simulink model "Copy_of_CM13_2024a_MachE_for_UA_HIL"  (R2024a)
settings: Solver=ode1  StartTime=0.0  StopTime=Inf  FixedStep=0.001  RelTol=1e-3  EnableMultiTasking=on
PreLoadFcn:
  | % if ~length(which('cmcmd')), cmenv; end
PostLoadFcn:
  | if any(exist('dsrtsu_mdlpostloadfcn', 'file') ~= 0), dsrtsu_mdlpostloadfcn('Execute', bdroot); end
InitFcn:
  | , if any(exist('rtifpga_mdlclblib', 'file') ~= 0), rtifpga_mdlclblib('Init', bdroot); end,
  | , if any(exist('dsmpb_private', 'file') ~= 0), dsmpb_private('dsmpb_mdlclblib', 'Init', bdroot); end,
undefined symbols (not defined in the file or in its folder): AccelCmd, ActTqLF_Nm_, ActTqLR_Nm_, ActTqRF_Nm_, ActTqRR_Nm_, BattChargeLimitMaxPwr, BattChargeLimitSocBpts, BattChargeLimitTbl, BattChrgCapcty, BattDischargeLimitSocBpts, BattDischargeLimitTbl, BattDischargeMaxPwr, BattNumCellsParallel, BattNumCellsSeries, BattOpenVoltCapBpts, BattOpenVoltTbl, BattResistSocBpts, BattResistTbl, BattResistTempBpts, BrakeMaxPrs, BrakeMaxTrq, ChassisDistCg2FrontAxle, ChassisDistCg2RearAxle, ChassisVehMass, CltchCmd, CoastDown, DecelCmd, DiffRatio, DiscIntNeverNeededParam, EnvGravCnst, EnvPrs, EnvTemp, FuelSpecificGrav, GearCmd, h, InitStates, lgSw, limitedMCT, MCT, MtrEffSpdBpts, MtrEffTbl, MtrEffTrqBpts, MtrPwrMax, MtrTrqMax, planned_speed, planned_time, pMCT, RealSimPara, ref_speed, Ref_speed, ref_time, Ref_time, rticanmm_blockfcn, rticanmm_initfcn, SteeringCmd, SupvsryCtrlRegenBrkCutOffTbl, SupvsryCtrlRegenSpdBpts, TestScnrioCycleNum, US06, VEH
libraries: simulink x264, VSIGenLib x262, etargetslib x201, dsmpblib x161, CarMaker4SL x142, rtimmsu_dsrtlib x32, vehdynlibtire x24, autolibshared x19, vehdynlibsuspension x14, vehdynlibtirecommon x14, autolibutils x10, VsrLibWheel x8
(part 5 of 47)

== system Copy_of_CM13_2024a_MachE_for_UA_HIL/Vehicle Under Test3/Environment ==
  Grade : Inport
  Friction : Constant  Value=ones(4,1).*1
  Ground Feedback : Subsystem  Variant=on  VariantControlMode=label  LabelModeActiveChoice=0
  Ground Z Level : Constant  Value=zeros(4,1)
  Subsystem : Subsystem
  Subsystem1 : Subsystem
      mask Display: disp('')
  Env : Outport
  wires:
  Subsystem/3(WindVel) -> Subsystem1/3(WindVel)
  Subsystem/2(EnvTemp) -> Subsystem1/2(EnvTemp)
  Subsystem/4(RoadGrade) -> Subsystem1/4(RoadGrade)
  Subsystem/1(EnvPrs) -> Subsystem1/1(EnvPrs)
  Subsystem1/1(Env) -> Env/1
  Friction/1 -> Ground Feedback/1(Friction)
  Ground Feedback/1(Ground) -> Subsystem1/5(GroundBus)  "Gnd"
  Ground Z Level/1 -> Ground Feedback/2(Ground Z Level)
  Grade/1 -> Subsystem/1(Grade)

== system Copy_of_CM13_2024a_MachE_for_UA_HIL/Vehicle Under Test3/Monitor ==
  Monitor : Inport
  Calculate Fuel MPG : Subsystem  Commented=on
  Calculate Powertrain Energy : Subsystem
  Terminator : Terminator
  Terminator3 : Terminator
  wires:
  Calculate Fuel MPG/1(FuelEconMPG) -> Terminator/1  "FuelEconMpg"
  Monitor/1 -> Calculate Powertrain Energy/1(Monitor), Calculate Fuel MPG/1(Monitor)
  Calculate Powertrain Energy/1(TransEnrgyOutkWh) -> Terminator3/1  "DiffEnrgyInkWh"

== system Copy_of_CM13_2024a_MachE_for_UA_HIL/Vehicle Under Test3/Performance Calculations ==
  VehSpd : Inport
  BattPwr : Inport  Port=2
  Divide : Product  Inputs=*/
  Divide1 : Product  Inputs=*/
  Divide2 : Product  Inputs=*/
  Integrator : Integrator
  Integrator1 : Integrator
  L/100 Km Calc : Product  Inputs=/*
  Product : Product
  Rate Transition3 : RateTransition  Deterministic=off
  Saturation : Saturate  UpperLimit=Inf  LowerLimit=0.001
  Saturation1 : Saturate  UpperLimit=Inf  LowerLimit=1e-3
  Sqrt : Sqrt
  US EPA kwh/USgal equivalent : Constant  Value=33.7
  US MPG Calc : Product  Inputs=*/
  m to 100Km : Gain  Gain=1/1000/100
  m to mile : Gain  Gain=0.000621371
  m^3 per gal : Gain  Gain=0.00378541
  m^3 to L : Gain  Gain=1000
  m^3 to US Gal : Gain  Gain=264.172
  s per h : Constant  Value=3600
  w per kw : Constant  Value=1000
  US MPG : Outport  VectorParamsAs1DForOutWhenUnconnected=off
  L/100Km : Outport  Port=2  VectorParamsAs1DForOutWhenUnconnected=off
  wires:
  VehSpd/1 -> Product/1, Product/2
  Product/1 -> Sqrt/1
  Sqrt/1 -> Integrator/1
  BattPwr/1 -> Divide/1
  US EPA kwh/USgal equivalent/1 -> Divide2/2
  m^3 per gal/1 -> Integrator1/1
  Divide1/1 -> m^3 per gal/1
  s per h/1 -> Divide1/2
  Divide2/1 -> Divide1/1
  Divide/1 -> Divide2/1
  w per kw/1 -> Divide/2
  Rate Transition3/1 -> US MPG/1  "US MPG"
  Saturation1/1 -> US MPG Calc/2
  US MPG Calc/1 -> Rate Transition3/1
  L/100 Km Calc/1 -> L/100Km/1  "L/100Km"
  m to 100Km/1 -> Saturation/1
  Saturation/1 -> L/100 Km Calc/1
  Integrator1/1 -> m^3 to L/1, m^3 to US Gal/1
  m to mile/1 -> US MPG Calc/1
  Integrator/1 -> m to 100Km/1, m to mile/1
  m^3 to L/1 -> L/100 Km Calc/2
  m^3 to US Gal/1 -> Saturation1/1

== system Copy_of_CM13_2024a_MachE_for_UA_HIL/Vehicle Under Test3/Vehicle ==
  note: With tire radius correction of 1.14
  note: NOT USED
  note: Vehicle simulation type:
      | 0- Simulink offline model
      | 1- Rototest HIL model
  note: NOT USED
  Env : Inport
  Driver : Inport  Port=2
  CarCmd : Inport  Port=3
  Abs : Abs  Commented=on  SaturateOnIntegerOverflow=off
  Actuation and Outputs : Subsystem
  AxT : Scope
  AxT2 : Scope  Commented=on
  Battery : Subsystem
  Bus Creator : BusCreator  Inputs=6
  Bus Selector : BusSelector  OutputSignals=Omega
  Bus Selector1 : BusSelector  Commented=on  OutputSignals=BRAKE_LAMP_BOOL_CAN,STEERING_ANGLE_DEG_CAN
  Bus Selector2 : BusSelector  Commented=on  OutputSignals=CarTrqT2W,VehSpd,Fx
  Bus Selector3 : BusSelector  Commented=on  OutputSignals=PT IF WFL rotv,PT IF WFR rotv,PT IF WRL rotv,PT IF WRR rotv
  Constant : Constant  Commented=on  Value=0  SampleTime=-1
  Data Type Conversion : DataTypeConversion  Commented=on  SaturateOnIntegerOverflow=off  RndMeth=Floor
  Data Type Conversion1 : DataTypeConversion  Commented=on  SaturateOnIntegerOverflow=off  RndMeth=Floor
  DriveCycle_trigger : Constant  Value=0
  Driver and Drive Cycle : Subsystem  TreatAsAtomicUnit=on
  From CAN : Subsystem  Commented=on
  From10 : From  Commented=on  GotoTag=VehSpdKph
  Front Wheel Drive : Subsystem  Variant=on  VariantControlMode=label  VariantControl=1  LabelModeActiveChoice=Choice
  Gain : Gain  Gain=3.6
  Gain1 : Gain  Commented=on  Gain=3.6*1.1414
  Goto10 : Goto  Commented=on  GotoTag=VehSpdKph
  Goto7 : Goto  Commented=on  GotoTag=BrakePressedCAN
  Goto8 : Goto  Commented=on  GotoTag=SteeringCAN
  Motor : Subsystem
  MtT : Scope
  MtT1 : Scope
  Multiport Switch : MultiPortSwitch  DataPortOrder=Zero-based contiguous  Inputs=2  zeroidx=on  SaturateOnIntegerOverflow=off  InputSameDT=off
  "Powertrain Supervisory Controller " : Subsystem  AncestorBlock=LibPtSupervisoryCtrl/Powertrain Supervisory Controller
  "Rototest UDP RX ExternalMode  " : Subsystem  Commented=on
  "Rototest UDP TX ExternalMode  " : Subsystem  Commented=on
  Rototest and ORNL Interface : Subsystem  Commented=on
  SUMO_speed_level : Constant  Value=0
  Scope : Scope
  Switch : Switch  Commented=on  Threshold=0.1  SaturateOnIntegerOverflow=off  InputSameDT=off
  Terminator{,1..2,4} (4 alike) : Terminator  Commented=on
  Terminator3 : Terminator
  To Workspace1 : ToWorkspace  VariableName=rotoOmega1  SampleTime=-1
      settings: Save2DSignal=2-D array (concatenate along first dimension)
  To Workspace2 : ToWorkspace  Commented=on  VariableName=rotoOmega  SampleTime=-1
      settings: Save2DSignal=2-D array (concatenate along first dimension)
  Transfer Fcn{,1..3} (4 alike) : TransferFcn  Commented=on  Denominator=[0.01 1]
  Transfer Fcn12 : TransferFcn  Commented=on  Denominator=[0.02 1]
  Vector Concatenate : Concatenate  Commented=on  NumInputs=4
  Vehicle Dynamics : Subsystem  Variant=on  VariantControlMode=label  LabelModeActiveChoice=Veh14DOF  mask{VehDynSel=Vehicle 14DOF}
      mask prompts: VehDynSel "Select the driver"
      mask init: same as Copy_of_CM13_2024a_MachE_for_UA_HIL/Vehicle Under Test2/Vehicle/Vehicle Dynamics
      mask TypeOptions VehDynSel: Vehicle Longitudinal | Vehicle 7DOF | Vehicle 14DOF
  VehicleSimulationType : Constant  Value=0
  omega : Scope
  Veh : Outport
  Output : Outport  Port=2
  wires:
  "Powertrain Supervisory Controller "/1(SupvsryCtrl) -> Vehicle Dynamics/2(SupvsryCtrl), Motor/1(SupvsryCtrl), [SupvsryCtrl]
  Driver/1 -> "Powertrain Supervisory Controller "/1(Driver)
  Bus Creator/1 -> Veh/1  "Veh"
  [SupvsryCtrl] -> Bus Creator/1  "SupvsryCtrl"
  [Batt] -> Bus Creator/2  "Batt"
  [Mtr] -> Bus Creator/3  "Mtr"
  [Whl] -> Bus Creator/5  "Whl"
  [Chassis] -> Bus Creator/6  "Chassis"
  Battery/1(Batt) -> [Batt], "Powertrain Supervisory Controller "/4(Batt)
  Motor/1(Mtr) -> "Powertrain Supervisory Controller "/3(Mtr), [Mtr]
  Env/1 -> Vehicle Dynamics/1(Env)
  Vehicle Dynamics/2(Chassis) -> "Powertrain Supervisory Controller "/2(Chassis), [Chassis]
  Vehicle Dynamics/1(Whl) -> [Whl]
  [Whl] -> Bus Selector/1
  [Diff] -> Bus Creator/4  "Diff"
  Front Wheel Drive/1(Diff) -> [Diff]
  Front Wheel Drive/3(PropShaftSpd) -> MtT1/1, Motor/2(MtrSpd)
  Motor/2(MtrTrq) -> Front Wheel Drive/1(DrvShfTrq), MtT/1
  Front Wheel Drive/2(AxlTrq) -> AxT/1, Vehicle Dynamics/3(AxlTrq)
  Rototest and ORNL Interface/2(Powertrain Out) -> Bus Selector3/1, Terminator/1
  Rototest and ORNL Interface/4(WhlSpd) -> To Workspace2/1, Terminator4/1  "WhlSpdCmd"
  Vehicle Dynamics/3(RototestInput) -> [RototestInput]
  VehicleSimulationType/1 -> Multiport Switch/1
  Driver and Drive Cycle/1(DriverBus) -> Actuation and Outputs/1(Driver Commands)
  Bus Selector1/1 -> Data Type Conversion1/1  "<BRAKE_LAMP_BOOL_CAN>"
  Data Type Conversion/1 -> Goto8/1  "SteerAngleCAN"
  "Rototest UDP RX ExternalMode  "/1(Data Vector) -> Rototest and ORNL Interface/2(UDP Input)
  Data Type Conversion1/1 -> Rototest and ORNL Interface/3(BRAKE_PRESSED), Goto7/1, Terminator2/1  "BrakePressed_flag"
  Bus Selector1/2 -> Data Type Conversion/1  "<STEERING_ANGLE_DEG_CAN>"
  From CAN/1(IO_Out) -> Bus Selector1/1
  Actuation and Outputs/1(BrakeSwitch) -> From CAN/1(BrakeSwitch)
  Actuation and Outputs/2(CAVE_Driver) -> Terminator3/1  "CAVE_Driver_Cmd"
  Rototest and ORNL Interface/3(DataSend) -> "Rototest UDP TX ExternalMode  "/1(Rototest_UDP_TX)  "Rototest_UDP_TX"
  Rototest and ORNL Interface/1(BrakeUpd) -> Terminator1/1
  [RototestInput] -> Bus Selector2/1
  Bus Selector2/3 -> Rototest and ORNL Interface/5(FXIN)  "<Fx>"
  Bus Selector2/2 -> Transfer Fcn12/1  "<VehSpd>"
  Bus Selector2/1 -> Rototest and ORNL Interface/1(CarTrqT2W)  "<CarTrqT2W>"
  Bus Selector/1 -> Multiport Switch/2  "<Omega>"
  Bus Selector3/1 -> Transfer Fcn/1  "<PT IF WFL rotv>"
  Bus Selector3/2 -> Transfer Fcn1/1  "<PT IF WFR rotv>"
  Bus Selector3/3 -> Transfer Fcn2/1  "<PT IF WRL rotv>"
  Bus Selector3/4 -> Transfer Fcn3/1  "<PT IF WRR rotv>"
  Vector Concatenate/1 -> Scope/1, To Workspace1/1, [OmegaRoto]
  [OmegaRoto] -> Multiport Switch/3
  Gain1/1 -> AxT2/1, Rototest and ORNL Interface/4(vehSpeedKph), Goto10/1  "VehSpdKph"
  Gain/1 -> Driver and Drive Cycle/1(Veh speed feedback [kph])
  DriveCycle_trigger/1 -> Driver and Drive Cycle/2(Veh speed cycle trigger)
  Multiport Switch/1 -> Front Wheel Drive/2(Omega), omega/1
  Constant/1 -> Switch/3
  Switch/1 -> Gain1/1
  Abs/1 -> Switch/2
  Transfer Fcn/1 -> Vector Concatenate/1
  Transfer Fcn1/1 -> Vector Concatenate/2
  Transfer Fcn2/1 -> Vector Concatenate/3
  Transfer Fcn3/1 -> Vector Concatenate/4
  Transfer Fcn12/1 -> Switch/1, Abs/1
  CarCmd/1 -> Actuation and Outputs/2(CarlaGBS), Driver and Drive Cycle/4(CarlaRef)
  Driver and Drive Cycle/2(Output) -> Output/1
  SUMO_speed_level/1 -> Driver and Drive Cycle/3(SUMO Veh speed Cmd Level)
  [vehSpeedSim] -> Gain/1
  connections:
  Battery/RConn1 -- Motor/LConn1

== system Copy_of_CM13_2024a_MachE_for_UA_HIL/CarMaker/IPG Vehicle/AEB Flag ==
  Bus Selector : BusSelector  OutputSignals=ACCDATA_2.CmbbBrkDecel_A_Rq,PowertrainData_10.TrnRng_D_Rq,PowertrainData_10.TrnPrkSys_D_Actl,PowertrainData_10.GearPos_D_Actl,PowertrainData_10.GearLvr_D_ActlDrv,Battery_Traction_2_FD1.BattTrac_U2_Actl,Battery_Traction_2_FD1.BattTrac_I2_Actl
  Gain{,1..4,6} (6 alike) : Gain
  RTICANMM ControllerSetup : Subsystem  InitFcn=rticanmm_blockfcn('InitFcn', 'CANnedySetup', gcb)  ClipboardFcn=rticanmm_blockfcn('ClipboardFcn', 'CANnedySetup', gcb)  mask(RTICANMM){DSProperties=struct('RTI',struct('Version',uint32(1),'BlockType',struct('isSLSource',uint8(1),'isSLSink',uint8(1),'isHWSource',uint8(0),'isHWSink',uint8(0),'isSetup',uint8(0),'isInline',uint8(1),'isNonInline',uint8(0),'isInterrupt',uint8(0),'isChannelwise',uint8(0)),'IOBoardType','RTICANMM','UnitType','RTICANMM','Identifier','BUSSETUP','DialogType','SL','BlockSet','RTICANMM','SlaveProcessor','CAN')), CANMMProperties=struct('cannedy',struct('data',struct('options',struct('controllername','MachE_FD1','controllernameautomatic',0,'loglevel','0','checkrealtime',0,'checkchangebaudrate',0,'sampletime','1.000','CANControllerStatus',1,'NumberofStuffErr',0,'NumberofFormErr',0,'NumberofAckErr',0,'NumberofBit0Err',1,'NumberofsuccrecRX',0,'Numberofsuccsent',0,'NumberofBit1Err',1,'NumberofCRCErr',1,'NumberoflostRX',0,'Busoff',0,'Busload',0,'OperationPending',0,'TxRetryCount',3,'addtrcexclusion',true,'cannavigator',struct('checkmonitoring',0,'checkinternmonitoring',0),'show_usrtrc',0,'use_usrtrc',0,'checkchangebaudrateFD',0,'errorframegeneration',0,'efgenabled',1),'modelroot','C:\GitDev\Yunli\FordMachE\HIL-Operation\src_cm4sl','generalsettings',struct('setupdata',struct('board','DS2671','boardno',1,'channelno',1,'Type','STD','transceiver',['ISO 11898-2 HIGH SPEED CAN'],'busconfig',[],'feedthrough','false','resistance',struct('r120',1,'roff',0,'r16',0,'r10',1),'baudrate','500','Frequency',[24 36],'samplemode',1,'commChannelTJA1041',6,'config',struct('standard',1,'advanced',0,'register',struct('btr0','0xC0','btr1','0x6F','sp','70','sjw','v','tseg1','15','tseg2','6','brp','0','smpl','0','btr0_36','0x1','btr1_36','0x2D','sp_36','83','sjw_36','0','tseg1_36','12','tseg2_36','2','brp_36','1','smpl_36','0','btr0_64','0x3','btr1_64','0x2B','sp_64','81','sjw_64','0','tseg1_64','11','tseg2_64','2','brp_64','3','smpl_64','0')),'channelcfg',struct('INTENDISABLE','CAN_INT_DISABLE','intenable',0),'SETUPID','RTICANMM_MachE_FD1_ID','CONTROLLER_ID','CANMM_CTL_SETUP_MachE_FD1','mainblock_includefile','RTICANMM_SETUP_MachE_FD1','canfdenable',2,'canfdboardselected',1,'slotno',1,'moduletype','DS4342','baudrateFD','2000','samplePoint','80','samplePointFD','80','termination','TERMINATION_ON'),'filesettings',struct('destfolder',struct('Name','RTICANMM_FILES','Check',1),'buildfolder',struct('Name','.','Check',1))),'advanced',struct('options',ones(1,100)),'partialnetdata',struct('switchedon',0,'format','STD','idmask',['XXXXX XXXXXXXX XXXXXXXX XXXXXXXX'],'idcode','0','idfilter','0','datamaskused',0,'datalength','0','datamask','0x0000000000000000','partialnetworkenable',0)),'blk',['HIL_MachE_CM10/Vehicle Under Test/Vehicle/AEB Flag/RTICANMM' char(10) 'ControllerSetup'],'allgeneratedfiles',{{'C:\GitDev\Yunli\FordMachE\HIL-Operation\src_cm4sl\RTICANMM_FILES\RTICANMM_SETUP_MachE_FD1.c','C:\GitDev\Yunli\FordMachE\HIL-Operation\src_cm4sl\RTICANMM_FILES\RTICANMM_SETUP_MachE_FD1.h','c:\gitdev\yunli\fordmache\hil-operation\src_cm4sl\rticanmm_files\rticanmm_setup_mache_fd1.mexw64'}},'ismp',false,'BlockDataVersion','0.9.0','recreate',0,'CANnedyTag','MachE_FD1'),'CANnedynew',0,'CANnedySettings','MachE_FD1','GeneratedFiles',{{'C:\GitDev\Yunli\FordMachE\HIL-Operation\src_cm4sl\RTICANMM_FILES\RTICANMM_SETUP_MachE_FD1.c','C:\GitDev\Yunli\FordMachE\HIL-Operation\src_cm4sl\RTICANMM_FILES\RTICANMM_SETUP_MachE_FD1.h','c:\gitdev\yunli\fordmache\hil-operation\src_cm4sl\rticanmm_files\rticanmm_setup_mache_fd1.mexw64'}},'SFCN','RTICANMM_SETUP_MachE_FD1.c','HostService',struct('Tags',struct('DATA','RTICANMM_MonitorData','TimeStampGlobal','RTICANMM_MonitoringTimeStamp','TimeStampGlobalEnable','RTICANMM_MonitoringTimeStampEnable','Enable','CANMMMonitor_MachE_FD1','TimeStamp','MonitoringTimeStamp_MachE_FD1'),'DATA',struct('Length',18),'Info',struct('Desc',{'ID','Service','Data1','Data2','Data3','Data4','Data5','Data6','Data7','Data8','Data9','Data10','Data11','Data12','Data13','Data14','Data15','Data16'}),'Names',struct('TimeStampGlobal','TimeStamp','TimeStampGlobalEnable','TimeStamp_Enable','Enable','Monitoring_Enable','TimeStamp','Monitoring_TimeStamp'),'ChannelID',2)), CANMMType=CANnedySetup, CANMMFolder=C:\CM_Projects\UA_cave\CM13_proj\src_cm4dspace_realsim, CANMMDestFolder=RTICANMM_FILES, CANMMSettings=MachE_FD1, CANMMSFcn=RTICANMM_SETUP_MachE_FD1, CANMMBoard=DS2671, CANMMBoardNum=1, CANMMChannel=1}
      settings: AttributesFormatString=%<CANMMSettings>  CopyFcn=rticanmm_blockfcn('CopyFcn', 'CANnedySetup', gcb)  DeleteFcn=rticanmm_blockfcn('DeleteFcn', 'CANnedySetup', gcb)  ModelCloseFcn=rticanmm_blockfcn('ModelCloseFcn', 'CANnedySetup', gcb)  NameChangeFcn=rticanmm_blockfcn('NameChangeFcn', 'CANnedySetup', gcb)  OpenFcn=try, rticanmm_setup_gui('create',gcb); ; catch,errordlg({lasterr, '','Please check your RTI installation.'},['Error: ' upper(bdroot)], 'replace'); end  MoveFcn=rticanmm_blockfcn('MoveFcn', 'CANnedySetup', gcb)
      mask Help: eval('rticanmm_quickstart(''create'', gcb);', 'disp(lasterr);')
      mask Display:
      | disp('RTI CAN\nMultiMessage\nControllerSetup')
      | 
      | port_label('input', 1 , 'Variation')
      | port_label('input', 2 , 'Reset')
      | port_label('output', 1, 'Status')
      | port_label('output', 2, 'Bit 0 errors')
      | port_label('output', 3, 'Bit 1 errors')
      | port_label('output', 4, 'CRC errors')
  RTICANMM ControllerSetup1 : dsmpblib/Data Outport  Priority=-10000
      settings: SourceProductName=dSPACE Model Interface Package for Simulink (MIPS)
  RTICANMM MainBlock : Subsystem  InitFcn=rticanmm_blockfcn('InitFcn', 'CANnedy', gcb)  ClipboardFcn=rticanmm_blockfcn('ClipboardFcn', 'CANnedy', gcb)  mask(RTICANMM){DSProperties=struct('RTI',struct('Version',uint32(1),'BlockType',struct('isSLSource',uint8(1),'isSLSink',uint8(1),'isHWSource',uint8(0),'isHWSink',uint8(0),'isSetup',uint8(0),'isInline',uint8(1),'isNonInline',uint8(0),'isInterrupt',uint8(0),'isChannelwise',uint8(0)),'IOBoardType','RTICANMM','UnitType','RTICANMM','Identifier','Mainblock','DialogType','SL','BlockSet','RTICANMM','SlaveProcessor','CAN')), CANMMProperties=struct('RTICANMMVersion','24.1','RTICANMMVersionIntern','24.1.739338.0305092592','RTICANMMDate','02-May-2024','Settings','RTICANMM_MAIN_MachE_FD1','UserTracePath','','ModelPath','C:\CM_Projects\UA_cave\CM13_proj\src_cm4dspace_realsim','filesettings',struct('FileName','RTICANMM_FILES\FD1_CAN_CX727_BEV_MY21_DCV_V21.dbc','IsRelative',1,'ClusterId',1,'ClusterList',{{'default'}},'destfolder',struct('Name','RTICANMM_FILES','Check',1),'buildfolder',struct('Name','.','Check',1),'onlyfreerawcapture',0,'overlapping2variant',0,'canfdsupport',1,'shortestJ2container',1),'onlyfreerawcapture',0,'Board','DS2671','BoardNum','1','ChannelNum','1','Variation','1','SetupId','MachE_FD1','MARK',['1F517A29CDDA91C40D81A06F1A259F';'402B427622E552C8724AFAF21BAF37';'507793A5241270CA8226E0AA5FABF0';'03D6615B00574698D00C6826B10C14';'3DF76DA45C804484AF6D3344981453'],'date','08-May-2025','clock',['08.05.2025 17:13:54'],'recreate',0,'RTIVER','DSRT','j1939',0,'TRC',struct('include',1),'rtsupport',struct('XMLFile','C:\CM_Projects\UA_cave\CM13_proj\src_cm4dspace_realsim\RTICANMM_FILES\RTICANMM_MAIN_MachE_FD1.xml','DBCXML',struct('Path','C:\CM_Projects\UA_cave\CM13_proj\src_cm4dspace_realsim\RTICANMM_FILES\RTICANMM_MAIN_MachE_FD1_dbc.xml','support',1,'Name','FD1_CAN_CX727_BEV_MY21_DCV_V21.dbc','Date',['28-Mar-2023 17:18:35'],'Type','CAN_FD','DBCSupport','ON'))), CANMMType=CANnedy, CANMMUserTraceMerged=off, CANMMUserTracePath=, CANMMChannelNum=1, CANMMBoardNum=1, CANMMDestFolder=RTICANMM_FILES, CANMMFolder=., CANMMSetupId=MachE_FD1, CANMMsave2mat=['1F517A29CDDA91C40D81A06F1A259F';'402B427622E552C8724AFAF21BAF37';'507793A5241270CA8226E0AA5FABF0';'03D6615B00574698D00C6826B10C14';'3DF76DA45C804484AF6D3344981453'], CANMMName=MachE_FD1, CANMMSettings=RTICANMM_MAIN_MachE_FD1, CANMMIntermediateTag=RTICANMM_MAIN_MachE_FD1_intermediate, CANMMsfcnname=RTICANMM_MAIN_MachE_FD1}
      mask init:
      | rticanmm_initfcn(gcb, CANMMType, CANMMsfcnname)
      settings: AttributesFormatString=MachE_FD1[MachE_FD1]  CopyFcn=rticanmm_blockfcn('CopyFcn', 'CANnedy', gcb)  DeleteFcn=rticanmm_blockfcn('DeleteFcn', 'CANnedy', gcb)  ModelCloseFcn=rticanmm_blockfcn('ModelCloseFcn', 'CANnedy', gcb)  NameChangeFcn=rticanmm_blockfcn('NameChangeFcn', 'CANnedy', gcb)  OpenFcn=try, rticanmm_main_gui('create',gcb); ; catch,errordlg({lasterr, '','Please check your RTI installation.'},['Error: ' upper(bdroot)], 'replace'); end  MoveFcn=rticanmm_blockfcn('MoveFcn', 'CANnedy', gcb)
      mask Help: try, rticanmm_quickstart('create', gcb); catch ME, disp(ME.message);end
      mask Display:
      | disp(sprintf('RTI CAN\nMultiMessage\nMainBlock'))
      | port_label('output', 1, 'RX Data')
  Reset@RTICANMM ControllerSetup : Constant  Value=0  OutDataTypeStr=boolean
  Terminator{,1..6,9..11} (10 alike) : Terminator
  Variation@RTICANMM ControllerSetup : Constant  OutDataTypeStr=uint8
  Output : Outport
  wires:
  Variation@RTICANMM ControllerSetup/1 -> RTICANMM ControllerSetup/1(VariationInput)
  Reset@RTICANMM ControllerSetup/1 -> RTICANMM ControllerSetup/2(Reset)
  Bus Selector/1 -> Output/1  "<CmbbBrkDecel_A_Rq>"
  Bus Selector/2 -> Gain4/1  "<TrnRng_D_Rq>"
  RTICANMM ControllerSetup/1(BUS_STATE) -> Terminator1/1  "FD1_status"
  RTICANMM ControllerSetup/2(STATUS_BIT0_ERROR) -> Terminator2/1  "FD1_bit0_err"
  RTICANMM ControllerSetup/3(STATUS_BIT1_ERROR) -> Terminator3/1  "FD1_bit1_err"
  RTICANMM ControllerSetup/4(STATUS_CRC_ERROR) -> Terminator4/1  "FD1_CRC_err"
  Bus Selector/3 -> Gain3/1  "<TrnPrkSys_D_Actl>"
  Bus Selector/6 -> Gain2/1  "<BattTrac_U2_Actl>"
  Bus Selector/7 -> Gain1/1  "<BattTrac_I2_Actl>"
  Bus Selector/4 -> Gain/1  "<GearPos_D_Actl>"
  Bus Selector/5 -> Gain6/1  "<GearLvr_D_ActlDrv>"
  Gain4/1 -> Terminator6/1  "GearPos_D_Actl"
  Gain3/1 -> Terminator5/1  "GearPos_D_Actl"
  Gain/1 -> Terminator/1  "GearPos_D_Actl"
  Gain6/1 -> Terminator11/1  "GearLvr_D_Actl"
  Gain2/1 -> Terminator10/1  "BattTrac_U2_Actl"
  Gain1/1 -> Terminator9/1  "BattTrac_I2_Actl"
  RTICANMM MainBlock/1(RX_Data) -> Bus Selector/1

== system Copy_of_CM13_2024a_MachE_for_UA_HIL/CarMaker/IPG Vehicle/Actuation and Outputs ==
  note: Notes: 11.12.2024
      | Increased the brake limite from 50 to 80
  note: CarMaker Driver's Brake value is too mall to hold the Mach-E when parking
      | Instead of default value, we change it to 40%
  note: Pedal Control Selection
      | 1. Manual input
      | Gas: percentage
      | Brake: percentage
      | 2. From Driver bus commands
      | 3. CM Driver
      | 4. 0
  note: Temp added an Soft_AEB for testing
  note: Detect Rising signal from M_SW_signal.
      | When SW is turned on, reset AEB flag
  note: Driver Commands are [0,100] for both pedal and brake
  Driver Commands : Inport
  CM Driver Commands : Inport  Port=2
  AEB Cmd : Inport  Port=3
  A_M_SW_Sig : Inport  Port=4
  Veh_spd : Inport  Port=5
  AEB Flag Control : Logic  Operator=OR  IconShape=distinctive  AllPortsSameDT=off  OutDataTypeStr=boolean
  AND : Logic  IconShape=distinctive  AllPortsSameDT=off  OutDataTypeStr=boolean
  APP : Constant  Value=0
  AR_limit : Saturate  UpperLimit=100  LowerLimit=0
  Add : Sum
  Add1 : Sum
  BR_command_0to100 : Constant  Value=0
  BR_limit : Saturate  UpperLimit=80  LowerLimit=0
  Bus Creator : BusCreator  Inputs=2
  Bus Selector : BusSelector  Commented=on  OutputSignals=VhclCtrl Gas
  Bus Selector1 : BusSelector  OutputSignals=AccelPedalCmd
  Bus Selector2 : BusSelector  Commented=on  OutputSignals=VhclCtrl Brake
  Bus Selector3 : BusSelector  OutputSignals=BrakePedalCmd
  Compare To Constant : simulink/Logic and Bit Operations/Compare To Constant  relop=>=  const=3  OutDataTypeStr=boolean
  Compare To Constant1 : simulink/Logic and Bit Operations/Compare To Constant  relop=<=  const=0.1  OutDataTypeStr=boolean  ZeroCross=off
  Compare To Constant2 : simulink/Logic and Bit Operations/Compare To Constant  relop=<=  const=0.01  OutDataTypeStr=boolean  ZeroCross=off
  Constant : Constant  Value=0
  Constant1 : Constant  Value=0
  Constant2 : Constant  Value=0
  Detect Rise Positive : simulink/Logic and Bit Operations/Detect Rise Positive  vinit=0  OutDataTypeStr=boolean
  Gain : Gain  Gain=-1
  Gain1 : Gain  Gain=100
  Gain2 : Gain  Gain=100
  MOOG Brake Actuator : Subsystem
  Memory : Memory
  Min threshold for Brake switch : Constant  Value=0
  Multiport Switch1 : MultiPortSwitch  Inputs=4  SaturateOnIntegerOverflow=off  InputSameDT=off
  Multiport Switch2 : MultiPortSwitch  Inputs=4  SaturateOnIntegerOverflow=off  InputSameDT=off
  Pedal Reset : Constant  Value=0
  Pedal Robot Control Selection : Constant  Value=2
  Relational Operator : RelationalOperator  Operator=>  OutDataTypeStr=boolean  InputSameDT=off
  Soft_AEB : Constant  Value=0
  Switch : Switch  Criteria=u2 > Threshold  SaturateOnIntegerOverflow=off  InputSameDT=off
  Switch1 : Switch  Criteria=u2 > Threshold  SaturateOnIntegerOverflow=off  InputSameDT=off
  Switch4 : Switch  Criteria=u2 > Threshold  SaturateOnIntegerOverflow=off  InputSameDT=off
  Terminator : Terminator
  Vehicle Accel Pedal Voltage Output : Subsystem
  bped2br_N1 : Lookup_n-D  NumberOfTableDimensions=1  BreakpointsForDimension1=[0 0.1 0.2 100]  Table=[0 0 25 100]  InternalRulePriority=Speed  RndMeth=Simplest
  standstill brake [0,100] : Constant  Value=0.4
  BrakeSwitch : Outport  VectorParamsAs1DForOutWhenUnconnected=off
  CAVE_Driver : Outport  Port=2
  AEB_IS_Triggered : Outport  Port=3
  tag scope: BrakeDriver=global, CarlaSteer=global, GasDriver=global
  wires:
  Multiport Switch1/1 -> AR_limit/1
  APP/1 -> Multiport Switch1/2
  Bus Selector1/1 -> Multiport Switch1/3  "<AccelPedalCmd>"
  Gain2/1 -> Multiport Switch1/4
  Multiport Switch2/1 -> BR_limit/1
  Gain1/1 -> Multiport Switch2/4
  Driver Commands/1 -> Bus Selector3/1, Bus Selector1/1
  Pedal Robot Control Selection/1 -> Multiport Switch1/1, Multiport Switch2/1
  BR_command_0to100/1 -> Multiport Switch2/2
  CM Driver Commands/1 -> Bus Selector2/1, Bus Selector/1
  Bus Selector3/1 -> Multiport Switch2/3  "<BrakePedalCmd>"
  Min threshold for Brake switch/1 -> Relational Operator/2
  Relational Operator/1 -> BrakeSwitch/1  "BrakeSwitch"
  Constant/1 -> Multiport Switch1/5
  Constant1/1 -> [CarlaSteer], Multiport Switch2/5
  Bus Creator/1 -> CAVE_Driver/1
  BR_limit/1 -> MOOG Brake Actuator/1(Brake Pedal command [%]), Bus Creator/2, [BrakeDriver], Relational Operator/1  "BrakePedalCmd_pct"
  Switch/1 -> Vehicle Accel Pedal Voltage Output/1(APP_pct), [GasDriver], Bus Creator/1  "AccelPedalCmd_pct"
  Constant2/1 -> Switch1/1, Switch/1
  AEB Cmd/1 -> Gain/1
  Add/1 -> Memory/1
  Compare To Constant/1 -> Add1/2
  AR_limit/1 -> Switch/3  "AccelPedalCmd_pct"
  Gain/1 -> Compare To Constant/1
  Switch1/1 -> Add/2  "AccelPedalCmd_pct"
  Pedal Reset/1 -> AEB Flag Control/2
  Memory/1 -> AEB_IS_Triggered/1, Switch/2, Switch1/3
  A_M_SW_Sig/1 -> Detect Rise Positive/1
  Detect Rise Positive/1 -> AEB Flag Control/1
  AEB Flag Control/1 -> Terminator/1, Switch1/2  "AEB Flag Control"
  Soft_AEB/1 -> Add1/1
  Add1/1 -> Add/1
  standstill brake [0,100]/1 -> Switch4/1
  Compare To Constant1/1 -> AND/2
  Bus Selector2/1 -> Switch4/3  "<VhclCtrl Brake>"
  Switch4/1 -> Gain1/1  "BrakePedalPos_pct"
  Veh_spd/1 -> Compare To Constant1/1
  Bus Selector/1 -> Compare To Constant2/1, Gain2/1  "<VhclCtrl Gas>"
  Compare To Constant2/1 -> AND/1
  AND/1 -> Switch4/2

== system Copy_of_CM13_2024a_MachE_for_UA_HIL/CarMaker/IPG Vehicle/Brake ==
  note: When replacing the entire braking system,
      | be sure to disable the IPG brake model by using the brake
      | model 'Model Manager off' in the vehicle GUI.
  note: <Your model here>
  note: <Your model here>
  VehicleSimulationType : Inport
  Sync_In : Inport  Port=2
  Brake.IF.In : Inport  Port=3
  VhclCtrl.Brake : Inport  Port=4
  VhclCtrl.BrakeUpd : Inport  Port=5
  Brake : S-Function  FunctionName=CM_Sfun  Parameters='Brake'  SFunctionDeploymentMode=off  EnableBusSupport=off
  BrakeUpd : S-Function  FunctionName=CM_Sfun  Parameters='BrakeUpd'  SFunctionDeploymentMode=off  EnableBusSupport=off
  BusCreator1 : BusCreator  Inputs=16
  CreateBus Vhcl.Wheel.PT : Subsystem
  Demux : Demux  Outputs=16
      settings: DisplayOption=none
  Switch : Switch  Criteria=u2 > Threshold  SaturateOnIntegerOverflow=off  InputSameDT=off
  Sync_Out : Outport  VectorParamsAs1DForOutWhenUnconnected=off
  Vhcl.Wheel.PT : Outport  Port=2  VectorParamsAs1DForOutWhenUnconnected=off
  wires:
  Demux/16 -> BusCreator1/16  "Brake IF Trq_DriveSrc_trg d3"
  Demux/15 -> BusCreator1/15  "Brake IF Trq_DriveSrc_trg d2"
  Demux/14 -> BusCreator1/14  "Brake IF Trq_DriveSrc_trg d1"
  Demux/13 -> BusCreator1/13  "Brake IF Trq_DriveSrc_trg d0"
  Demux/12 -> BusCreator1/12  "Brake IF Trq_Reg_trg RR"
  Demux/11 -> BusCreator1/11  "Brake IF Trq_Reg_trg RL"
  Demux/10 -> BusCreator1/10  "Brake IF Trq_Reg_trg FR"
  Demux/9 -> BusCreator1/9  "Brake IF Trq_Reg_trg FL"
  Demux/8 -> BusCreator1/8  "Brake IF Trq_PB RR"
  Demux/7 -> BusCreator1/7  "Brake IF Trq_PB RL"
  Demux/6 -> BusCreator1/6  "Brake IF Trq_PB FR"
  Demux/5 -> BusCreator1/5  "Brake IF Trq_PB FL"
  Demux/4 -> BusCreator1/4  "Brake IF Trq_WB RR"
  Demux/3 -> BusCreator1/3  "Brake IF Trq_WB RL"
  Demux/2 -> BusCreator1/2  "Brake IF Trq_WB FR"
  Demux/1 -> BusCreator1/1  "Brake IF Trq_WB FL"
  Brake/2 -> Demux/1
  BrakeUpd/1 -> Sync_Out/1
  Brake/1 -> BrakeUpd/1  "Sync"
  Brake.IF.In/1 -> Brake/2
  VhclCtrl.Brake/1 -> Brake/3
  Sync_In/1 -> Brake/1
  BrakeUpd/2 -> CreateBus Vhcl.Wheel.PT/1(In)
  CreateBus Vhcl.Wheel.PT/1(Out) -> Vhcl.Wheel.PT/1
  VehicleSimulationType/1 -> Switch/2
  Switch/1 -> BrakeUpd/2
  BusCreator1/1 -> Switch/3
  VhclCtrl.BrakeUpd/1 -> Switch/1

== system Copy_of_CM13_2024a_MachE_for_UA_HIL/CarMaker/IPG Vehicle/CarAndTrailer ==
  Sync_In : Inport
  VhclCtrl.Steering : Inport  Port=2
  Vhcl.Wheel.In : Inport  Port=3
  Vhcl.Misc : Inport  Port=4
  CarAndTrailerUpd : Subsystem
  Forces : Subsystem
  Ground : Ground
  Kinematics : Subsystem
  Kinetics : Subsystem
  Steering : Subsystem
  Terminator : Terminator
  Terminator1 : Terminator
  Trailer : Subsystem
  Sync_Out : Outport  VectorParamsAs1DForOutWhenUnconnected=off
  Brake.IF.In : Outport  Port=2  VectorParamsAs1DForOutWhenUnconnected=off
  Car.Trq_T2W : Outport  Port=3
  wires:
  Trailer/9(Car.Hitch.FrcTrq) -> CarAndTrailerUpd/9(Car.Hitch.FrcTrq)
  Trailer/8(Vhcl.Wheel.RR) -> CarAndTrailerUpd/8(Vhcl.Wheel.RR)
  Trailer/7(Vhcl.Wheel.RL) -> CarAndTrailerUpd/7(Vhcl.Wheel.RL)
  Trailer/6(Vhcl.Wheel.FR) -> CarAndTrailerUpd/6(Vhcl.Wheel.FR)
  Trailer/5(Vhcl.Wheel.FL) -> CarAndTrailerUpd/5(Vhcl.Wheel.FL)
  Trailer/4(Vhcl.PoI) -> CarAndTrailerUpd/4(Vhcl.PoI)
  Trailer/3(Vhcl.Motion) -> CarAndTrailerUpd/3(Vhcl.Motion)
  Trailer/2(Vhcl.Steering) -> CarAndTrailerUpd/2(Vhcl.Steering)
  Trailer/1(Sync_Out) -> CarAndTrailerUpd/1(Sync_In)
  CarAndTrailerUpd/2(Brake.IF.In) -> Brake.IF.In/1
  CarAndTrailerUpd/1(Sync_Out) -> Sync_Out/1
  Vhcl.Misc/1 -> Terminator1/1
  Vhcl.Wheel.In/1 -> Terminator/1
  Kinetics/6(WheelCarrier.Misc) -> Trailer/6(WheelCarrier.Misc)
  Kinetics/5(Car.Trq_T2W) -> Car.Trq_T2W/1, Trailer/5(Car.Trq_T2W)
  Steering/2(Steer.IF) -> Kinematics/2(Steer.IF)
  Kinetics/4(Car.Fr1) -> Trailer/4(Car.Fr1)
  Kinetics/3(Car.Hitch) -> Trailer/3(Car.Hitch)
  Kinetics/2(Trailer.Load) -> Trailer/2(Trailer.Load)
  VhclCtrl.Steering/1 -> Steering/2(VhclCtrl.Steering)
  Sync_In/1 -> Steering/1(Sync_In)
  Steering/1(Sync_Out) -> Kinematics/1(Sync_In)
  Kinetics/1(Sync_Out) -> Trailer/1(Sync_In)
  Ground/1 -> CarAndTrailerUpd/10(Vhcl.Fr1A)
  Forces/11(FStabi_ext) -> Kinetics/11(FStabi_ext)
  Forces/10(FDamp_ext) -> Kinetics/10(FDamp_ext)
  Forces/9(FSpring_ext) -> Kinetics/9(FSpring_ext)
  Forces/8(TireRR_Out) -> Kinetics/8(TireRR.Out)
  Forces/7(TireRL_Out) -> Kinetics/7(TireRL.Out)
  Forces/6(TireFR_Out) -> Kinetics/6(TireFR.Out)
  Forces/5(TireFL_Out) -> Kinetics/5(TireFL.Out)
  Forces/4(Car.Load) -> Kinetics/4(Car.Load)
  Forces/2(Car.Virtual) -> Kinetics/2(Car.Virtual)
  Kinematics/6(lSpring) -> Forces/6(lSpring)
  Kinematics/7(vDamp) -> Forces/7(vDamp)
  Forces/3(Car.Aero) -> Kinetics/3(Car.Aero)
  Forces/1(Sync_Out) -> Kinetics/1(Sync_In)
  Kinematics/5(TireRR_In) -> Forces/5(TireRR_In)
  Kinematics/4(TireRL_In) -> Forces/4(TireRL_In)
  Kinematics/3(TireFR_In) -> Forces/3(TireFR_In)
  Kinematics/2(TireFL_In) -> Forces/2(TireFL_In)
  Kinematics/1(Sync_Out) -> Forces/1(Sync_In)
  Kinematics/8(lStabi) -> Forces/8(lStabi)
  Forces/12(FBuf_ext) -> Kinetics/12(FBuf_ext)
  Kinematics/9(lBuf) -> Forces/9(lBuf)

== system Copy_of_CM13_2024a_MachE_for_UA_HIL/CarMaker/IPG Vehicle/DARTS ConfigDesk Control ==
  Enable : Inport
  Range : Inport  Port=2
  Speed : Inport  Port=3
  Gain : Inport  Port=4
  Bus Creator : BusCreator  Inputs=4
  Bus Creator1 : BusCreator  Inputs=3
  Bus Creator2 : BusCreator  Inputs=3
  Bus Selector1 : BusSelector  OutputSignals=Range,Speed,Gain
  Constant : Constant  Value=77.0
  Constant1 : Constant  Value=1.0
  Constant11 : Constant  Value=0.0
  Constant12 : Constant  Value=0.0
  Constant2 : Constant  Value=0.52
  Constant3 : Constant  Value=13.0
  Constant4 : Constant  Value=13.0
  Constant5 : Constant  Value=0.3
  Constant6 : Constant  Value=0.0
  DARTS Eth : dsmpblib/Data Inport  Priority=10000
      settings: SourceProductName=dSPACE Model Interface Package for Simulink (MIPS)
  Demux : Demux  Outputs=3
  Demux1 : Demux  Outputs=3
  Ground : Ground
  Mux1 : Mux  Inputs=3
  Mux2 : Mux  Inputs=3
  Setup Status [DARTS Control (1)] : dsmpblib/Data Inport  Priority=10000
      settings: SourceProductName=dSPACE Model Interface Package for Simulink (MIPS)
  Setup [DARTS Control (1)] : dsmpblib/Data Outport  Priority=-10000
      settings: SourceProductName=dSPACE Model Interface Package for Simulink (MIPS)
  Status [DARTS Control (1)] : dsmpblib/Data Inport  Priority=10000
      settings: SourceProductName=dSPACE Model Interface Package for Simulink (MIPS)
  Targets Status [DARTS Control (1)] : dsmpblib/Data Inport  Priority=10000
      settings: SourceProductName=dSPACE Model Interface Package for Simulink (MIPS)
  Targets [DARTS Control (1)] : dsmpblib/Data Outport  Priority=-10000
      settings: SourceProductName=dSPACE Model Interface Package for Simulink (MIPS)
  Terminator{1..17} (17 alike) : Terminator
  Trigger [DARTS Control (1)] : dsmpblib/Data Outport  Priority=-10000
      settings: SourceProductName=dSPACE Model Interface Package for Simulink (MIPS)
  tag scope: dartsInput=global, dartsResponse=global
  wires:
  Setup Status [DARTS Control (1)]/9 -> Terminator10/1
  Ground/1 -> Trigger [DARTS Control (1)]/3, Trigger [DARTS Control (1)]/2, Trigger [DARTS Control (1)]/1
  Setup Status [DARTS Control (1)]/2 -> Terminator3/1
  Setup Status [DARTS Control (1)]/8 -> Terminator9/1
  Setup Status [DARTS Control (1)]/3 -> Terminator4/1
  Status [DARTS Control (1)]/1 -> Terminator11/1
  Setup Status [DARTS Control (1)]/6 -> Terminator7/1
  Setup Status [DARTS Control (1)]/5 -> Terminator6/1
  Setup Status [DARTS Control (1)]/7 -> Terminator8/1
  Setup Status [DARTS Control (1)]/4 -> Terminator5/1
  Status [DARTS Control (1)]/7 -> Terminator16/1
  Setup Status [DARTS Control (1)]/1 -> Terminator2/1
  Demux1/3 -> Bus Creator2/3  "OutGain"
  Status [DARTS Control (1)]/4 -> Terminator17/1
  Status [DARTS Control (1)]/5 -> Terminator14/1
  Bus Selector1/3 -> Mux2/3  "<Gain>"
  Status [DARTS Control (1)]/6 -> Terminator15/1
  Status [DARTS Control (1)]/2 -> Terminator12/1
  Constant11/1 -> Setup [DARTS Control (1)]/6
  Status [DARTS Control (1)]/3 -> Terminator13/1
  Mux2/1 -> Demux1/1
  Demux1/2 -> Bus Creator2/2  "OutSpeed"
  Demux1/1 -> Bus Creator2/1  "OutRange"
  Bus Selector1/2 -> Mux2/2  "<Speed>"
  Constant12/1 -> Setup [DARTS Control (1)]/2
  Constant/1 -> Setup [DARTS Control (1)]/1
  Bus Creator2/1 -> [dartsResponse]
  Constant4/1 -> Setup [DARTS Control (1)]/9
  Constant1/1 -> Setup [DARTS Control (1)]/5
  Constant6/1 -> Setup [DARTS Control (1)]/3
  Bus Selector1/1 -> Mux2/1  "<Range>"
  Constant2/1 -> Setup [DARTS Control (1)]/4
  DARTS Eth/1 -> Terminator1/1
  Constant3/1 -> Setup [DARTS Control (1)]/8
  Targets Status [DARTS Control (1)]/1 -> Bus Selector1/1
  Constant5/1 -> Setup [DARTS Control (1)]/7
  Demux/1 -> Bus Creator1/1  "InRange"
  Mux1/1 -> Demux/1
  Demux/3 -> Bus Creator1/3  "InGain"
  Bus Creator/1 -> Targets [DARTS Control (1)]/1
  Demux/2 -> Bus Creator1/2  "InSpeed"
  Bus Creator1/1 -> [dartsInput]
  Enable/1 -> Bus Creator/1  "Enable"
  Range/1 -> Mux1/1, Bus Creator/2  "Range"
  Speed/1 -> Mux1/2, Bus Creator/3  "Speed"
  Gain/1 -> Mux1/3, Bus Creator/4  "Gain"

== system Copy_of_CM13_2024a_MachE_for_UA_HIL/CarMaker/IPG Vehicle/Driver and Drive Cycle ==
  note: Rate Limiter note:
      | wet ground test: 7, -9.8
      | Ford default 5, -5
  note: Traffic light index:
      | Scenario based hack
      | 4,190,316 for UA road, route:Left lane straite
  note: Traffic light state/phase (integer):
      | 0: All lights off
      | 1: Green light on
      | 2: Yellow light on
      | 3: Red light on
      | 4: Red-Yellow light on
  note: Camera object type (integer)
      | 0 - Car
      | 1 - Truck
      | 2 - Bicycle
      | 3 - Pedestrian
      | 4 - Traffic sign
      | 5 - Traffic light
  note: DriveCycle temp comment out
  note: This selector in ControlDesk:
      | BYPASS CONTROLS -> ManSpdSel
      | Manual input in km/h
      | #Temp disabledl, 0 Speed
      | Speed from a IDM
      | Read from CM testrun file (this is for CRADA project automation)
      | 5. Speed from eco-driving history
      | 6. Zero speed
  Veh speed feedback [kph] : Inport
  Veh speed cycle trigger : Inport  Port=2
  AEB_IS_Triggered : Inport  Port=3
  "Auto_M_SW_Sig " : Inport  Port=4
  SUMO_spd : Inport  Port=5
  CM_Time : Inport  Port=6
  VehSpdRef : Inport  Port=7
  Add : Sum
  Add1 : Sum  Commented=on  Inputs=+-
  Add2 : Sum  Commented=on
  Add3 : Sum  Commented=on  Inputs=+-
  Automation_Spd_selection : Subsystem  Commented=on
  Automation_spd : Terminator
  Automation_spd1 : Terminator
  Bus Selector2 : BusSelector  Commented=on  OutputSignals=ObjID,Type,LightState
  CM state : Scope  Commented=on
  CM_drv_act_kmh : Scope  Commented=on
  Cam_obj_index : Constant  Commented=on  Value=0
  Camera Sensor Object : CarMaker4SL/Sensors/Camera Sensor Object  Commented=on  xname=1  xstime=Continuous
      settings: SourceProductName=CarMaker4SL
  CarV_kmh : Scope  Commented=on
  CaraX_ ms2 : Scope  Commented=on
  Clock{1..4} (4 alike) : Clock  Commented=on
  CoastDown : Lookup_n-D  Commented=through  NumberOfTableDimensions=1  BreakpointsForDimension1=CoastDown.Time  Table=CoastDown.Speed  InternalRulePriority=Speed  RndMeth=Simplest
  Compare To Constant : simulink/Logic and Bit Operations/Compare To Constant  Commented=on  relop===  const=8  OutDataTypeStr=boolean
  Constant : Constant  Value=6
  Constant1 : Constant  Value=0
  Constant2 : Constant  Value=5
  Constant3 : Constant  Value=0
  Constant4 : Constant  Commented=on  Value=0
  Data Type Conversion11 : DataTypeConversion  OutDataTypeStr=double  SaturateOnIntegerOverflow=off  RndMeth=Floor  LockScale=on
  Dis2lead_IPGdriver : Scope  Commented=on
  DriveCycleSelect : Constant
  Driver and PI with FF Control : Subsystem
  From4 : From  Commented=on  GotoTag=VehSpdRef  TagVisibility=global
  Gain : Gain  Gain=1/1.609
  Gain1 : Gain  Gain=1/1.609
  Gain2 : Gain  Gain=3.6
  Gain3 : Gain  Gain=3.6
  Gain4 : Gain  Commented=on  Gain=3.6
  Gain5 : Gain  Commented=on  Gain=3.6
  Gain6 : Gain  Commented=on  Gain=1.609
  Gain7 : Gain  Commented=on  Gain=1.609
  Get Cycle Clock Time : Subsystem  Commented=through
  IDM : Subsystem  Commented=on
  IDM Rate Limiter : RateLimiter  RisingSlewLimit=1.2  FallingSlewLimit=-6.5  SampleTimeMode=inherited
  Jinghui planned speed : Lookup_n-D  Commented=on  NumberOfTableDimensions=1  BreakpointsForDimension1=planned_time  Table=planned_speed  InternalRulePriority=Speed  RndMeth=Simplest
  LightState : Scope  Commented=on
  MCT : Lookup_n-D  Commented=through  NumberOfTableDimensions=1  BreakpointsForDimension1=MCT.Time  Table=MCT.Speed  InternalRulePriority=Speed  RndMeth=Simplest
  ManSpd : Constant  Value=0
  ManSpdSel : Constant
  Maxkmh_limiter : Saturate  UpperLimit=120  LowerLimit=0
  Memory1 : Memory  Commented=on
  Memory2 : Memory  Commented=on
  Minus : Sum  Commented=on  Inputs=+-
  Minus1 : Sum  Commented=on  Inputs=+-
  Multiport Switch : MultiPortSwitch  Inputs=5  SaturateOnIntegerOverflow=off  InputSameDT=off
  Multiport Switch1 : MultiPortSwitch  Inputs=7  SaturateOnIntegerOverflow=off  InputSameDT=off
  ObjectIndex : Scope  Commented=on
  Rate Limiter : RateLimiter  RisingSlewLimit=5  FallingSlewLimit=-5  SampleTimeMode=inherited
  Rate Limiter1 : RateLimiter  RisingSlewLimit=5  FallingSlewLimit=-5  SampleTimeMode=inherited
  Read CM Dict : CarMaker4SL/Read CM Dict  Commented=on  xname=SC.State  xsync=off  xstime=Continuous
  Read CM Dict1 : CarMaker4SL/Read CM Dict  Commented=on  xname=Car.ax  xsync=off  xstime=Continuous
  Read CM Dict2 : CarMaker4SL/Read CM Dict  Commented=on  xname=Driver.ReCon.Speed  xsync=off  xstime=Continuous
  Read CM Dict3 : CarMaker4SL/Read CM Dict  Commented=on  xname=Driver.Long.dv  xsync=off  xstime=Continuous
  Read CM Dict4 : CarMaker4SL/Read CM Dict  Commented=on  xname=Driver.ReCon.Trf_FOL.dDist  xsync=off  xstime=Continuous
  Read CM Dict5 : CarMaker4SL/Read CM Dict  Commented=on  xname=Car.v  xsync=off  xstime=Continuous
  Switch : Switch  Commented=on  Criteria=u2 ~= 0  SaturateOnIntegerOverflow=off  InputSameDT=off
  Switch1 : Switch  Commented=on  SaturateOnIntegerOverflow=off  InputSameDT=off
  Switch2 : Switch  Commented=on  SaturateOnIntegerOverflow=off  InputSameDT=off
  Terminator : Terminator
  Terminator1 : Terminator
  Terminator2 : Terminator  Commented=on
  Terminator3 : Terminator  Commented=on
  Terminator4 : Terminator
  US06 : Lookup_n-D  Commented=through  NumberOfTableDimensions=1  BreakpointsForDimension1=US06.Time  Table=US06.Speed  InternalRulePriority=Speed  RndMeth=Simplest
  driver look ahead seconds : Constant  Value=0.5
  limitedMCT : Lookup_n-D  Commented=through  NumberOfTableDimensions=1  BreakpointsForDimension1=limitedMCT.Time  Table=limitedMCT.Speed  InternalRulePriority=Speed  RndMeth=Simplest
  pMCT : Lookup_n-D  Commented=through  NumberOfTableDimensions=1  BreakpointsForDimension1=pMCT.Time  Table=pMCT.Speed  InternalRulePriority=Speed  RndMeth=Simplest
  real veh speed : Lookup_n-D  Commented=on  NumberOfTableDimensions=1  BreakpointsForDimension1=ref_time  Table=ref_speed  InternalRulePriority=Speed  RndMeth=Simplest
  DriverBus : Outport
  wires:
  Veh speed cycle trigger/1 -> Get Cycle Clock Time/1(Cycle Trigger)
  MCT/1 -> Multiport Switch/5
  US06/1 -> Multiport Switch/4
  Add/1 -> CoastDown/1, pMCT/1, limitedMCT/1, MCT/1, US06/1
  CoastDown/1 -> Multiport Switch/2
  pMCT/1 -> Multiport Switch/3
  DriveCycleSelect/1 -> Multiport Switch/1
  [VehSpdKph] -> Data Type Conversion11/1
  Driver and PI with FF Control/1(DriverBus) -> DriverBus/1
  Data Type Conversion11/1 -> Gain/1, Driver and PI with FF Control/1(Vehicle_Spd_kph)  "Vehicle_Spd_kph"
  Get Cycle Clock Time/1(tCycle) -> Add/2
  driver look ahead seconds/1 -> Add/1
  limitedMCT/1 -> Multiport Switch/6
  Veh speed feedback [kph]/1 -> [VehSpdKph]
  Gain/1 -> Terminator/1  "Vehicle_Spd_mph"
  Gain1/1 -> Terminator1/1  "Vehicle_SpdDmd_mph"
  ManSpd/1 -> Rate Limiter/1
  Rate Limiter/1 -> Multiport Switch1/2
  Multiport Switch/1 -> Automation_spd1/1
  Constant1/1 -> Multiport Switch1/8
  Automation_Spd_selection/1(Spd) -> Rate Limiter1/1, Automation_spd/1  "Automation_spd"
  AEB_IS_Triggered/1 -> Automation_Spd_selection/1(AEB_IS_Triggered)
  "Auto_M_SW_Sig "/1 -> Automation_Spd_selection/2(A_M_SW_sig)
  Rate Limiter1/1 -> Multiport Switch1/5
  SUMO_spd/1 -> Terminator4/1
  Gain2/1 -> Multiport Switch1/3  "Vehicle_SpdDmd_kmh"
  Read CM Dict4/1 -> Dis2lead_IPGdriver/1  "Trf_FOL_dDist"
  Gain3/1 -> Maxkmh_limiter/1  "Vehicle_SpdDmd_kmh"
  Maxkmh_limiter/1 -> Multiport Switch1/4
  Read CM Dict2/1 -> Add2/1
  Read CM Dict3/1 -> Gain4/1
  Gain4/1 -> Add2/2
  Read CM Dict5/1 -> Gain5/1  "VehSpd"
  Gain5/1 -> CarV_kmh/1
  Add2/1 -> CM_drv_act_kmh/1
  Camera Sensor Object/2 -> Bus Selector2/1
  Bus Selector2/1 -> Terminator2/1  "<ObjID>"
  Bus Selector2/2 -> Terminator3/1  "<Type>"
  Bus Selector2/3 -> LightState/1  "<LightState>"
  Cam_obj_index/1 -> Camera Sensor Object/2
  Camera Sensor Object/1 -> ObjectIndex/1
  Read CM Dict1/1 -> CaraX_ ms2/1  "VehSpd"
  CM_Time/1 -> IDM/1(CM_Time)
  Clock3/1 -> Add1/1
  ManSpdSel/1 -> Minus/1, Minus1/1, Multiport Switch1/1
  real veh speed/1 -> Gain6/1
  Clock2/1 -> Switch2/3
  Memory1/1 -> Switch2/1
  Add1/1 -> real veh speed/1  "tCycle"
  Switch2/1 -> Add1/2, Memory1/1
  Gain6/1 -> Multiport Switch1/6  "realV"
  Clock1/1 -> Switch1/3
  Add3/1 -> Jinghui planned speed/1  "tCycle"
  Memory2/1 -> Switch1/1
  Switch1/1 -> Add3/2, Memory2/1
  Clock4/1 -> Add3/1
  Jinghui planned speed/1 -> Gain7/1
  Gain7/1 -> Multiport Switch1/7  "refV"
  Constant/1 -> Minus/2
  Minus/1 -> Switch1/2
  Constant2/1 -> Minus1/2
  Minus1/1 -> Switch2/2
  Constant3/1 -> Gain2/1
  Multiport Switch1/1 -> Gain1/1, Driver and PI with FF Control/2(Vehicle_SpdDmd_kph)  "RefSpd [km/hr]"
  Read CM Dict/1 -> CM state/1, Compare To Constant/1
  Constant4/1 -> Switch/3
  Compare To Constant/1 -> Switch/2
  IDM Rate Limiter/1 -> Gain3/1
  VehSpdRef/1 -> IDM Rate Limiter/1

== system Copy_of_CM13_2024a_MachE_for_UA_HIL/CarMaker/IPG Vehicle/FD1 ==
  Bus Selector : BusSelector  OutputSignals=Simulated ECUs.FD1_CAN_P702_BEV_MY22_DCV_v12_06-7-2021.FD1_CAN_HCM.RX.PDUs.Body_Info_10_FD1.PosLghtFr_D_Stat.ISignal Value.GearRvrse_D_Actl Value,Simulated ECUs.FD1_CAN_P702_BEV_MY22_DCV_v12_06-7-2021.FD1_CAN_HCM.RX.PDUs.PowertrainData_10.TrnRng_D_Rq.ISignal Value.TrnRng_D_Rq Value,Simulated ECUs.FD1_CAN_P702_BEV_MY22_DCV_v12_06-7-2021.FD1_CAN_HCM.RX.PDUs.PowertrainData_10.TrnPrkSys_D_Actl.ISignal Value.TrnPrkSys_D_Actl Value,Simulated ECUs.FD1_CAN_P702_BEV_MY22_DCV_v12_06-7-2021.FD1_CAN_HCM.RX.PDUs.PowertrainData_10.GearLvr_D_ActlDrv.ISignal Value.GearLvr_D_ActlDrv Value,Simulated ECUs.FD1_CAN_P702_BEV_MY22_DCV_v12_06-7-2021.FD1_CAN_HCM.RX.PDUs.PowertrainData_10.GearPos_D_Actl.ISignal Value.GearPos_D_Actl Value
  MachE_CANConfig_In : dsmpblib/Data Inport  Priority=10000
      settings: SourceProductName=dSPACE Model Interface Package for Simulink (MIPS)
  Terminator{,8..9,14..15} (5 alike) : Terminator
  wires:
  Bus Selector/2 -> Terminator8/1  "<TrnRng_D_Rq Value>"
  MachE_CANConfig_In/1 -> Bus Selector/1
  Bus Selector/1 -> Terminator/1  "<GearRvrse_D_Actl Value>"
  Bus Selector/3 -> Terminator9/1  "<TrnPrkSys_D_Actl Value>"
  Bus Selector/5 -> Terminator15/1  "<GearPos_D_Actl Value>"
  Bus Selector/4 -> Terminator14/1  "<GearLvr_D_ActlDrv Value>"

== system Copy_of_CM13_2024a_MachE_for_UA_HIL/CarMaker/IPG Vehicle/From CAN ==
  Steering_ang_deg : Inport
  BrakeSwitch : Inport  Port=2
  Brake switch ource selection : Constant  Value=2
  Bus Creator1 : BusCreator  Inputs=2
  Demux : Demux  Outputs=1
  Ground1 : Ground
  Multiport Switch1 : MultiPortSwitch  Inputs=2  SaturateOnIntegerOverflow=off  InputSameDT=off
  IO_Out : Outport
  wires:
  Bus Creator1/1 -> IO_Out/1  "IO_Out"
  Multiport Switch1/1 -> Bus Creator1/2  "BRAKE_LAMP_BOOL_CAN"
  Demux/1 -> Bus Creator1/1  "STEERING_ANGLE_DEG_CAN"
  Steering_ang_deg/1 -> Demux/1
  Brake switch ource selection/1 -> Multiport Switch1/1
  Ground1/1 -> Multiport Switch1/2  "Brake switch from CAN"
  BrakeSwitch/1 -> Multiport Switch1/3
